simulink model "Speed_control"  (R2023a)
settings: Solver=VariableStepAuto  StartTime=0.0  StopTime=10.0  RelTol=1e-3
libraries: spsMosfetLib x6, simulink x6, spsControlledVoltageSourceLib x1
settings Model: Creator=SIDDHARTHI  LastModifiedBy=SIDDHARTHI

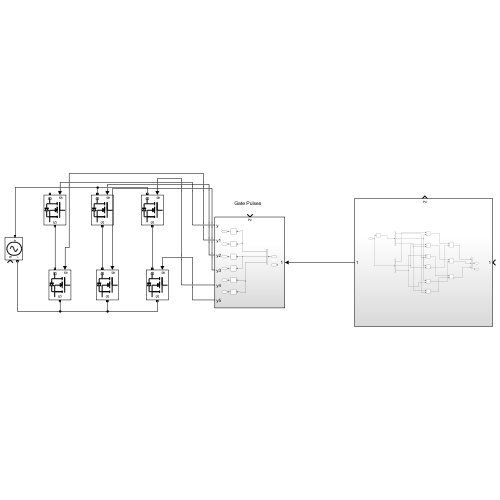
[thumbnail: Simulink's stored preview of the top-level diagram]
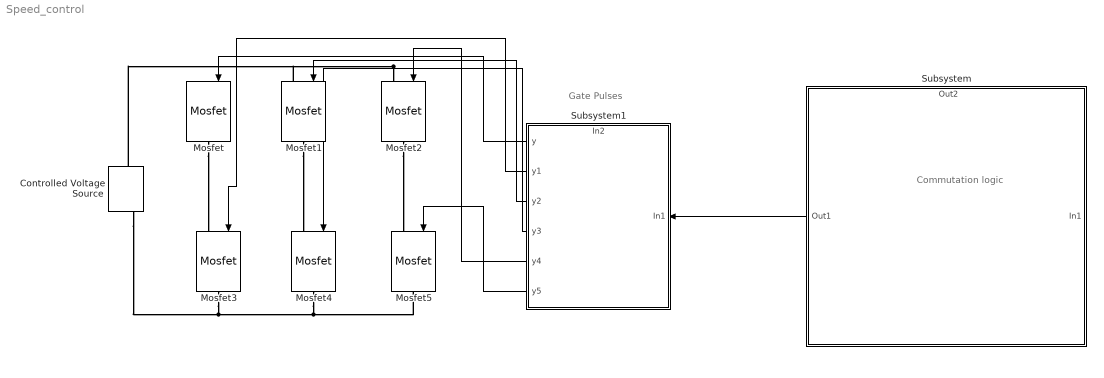
== system Speed_control ==
  note: Gate Pulses
  note: Commutation logic
  Controlled Voltage Source : spsControlledVoltageSourceLib/Controlled Voltage Source  Initialize=on  Source_Type=AC  Amplitude=0  Phase=0  Frequency=0  Measurements=None
  Mosfet{,1..5} (6 alike) : spsMosfetLib/Mosfet  Ron=0.1  Lon=0  Rd=0.01  Vfd=0  IC=0  Rs=1e5  Cs=inf  Measurements=off
  Subsystem : Subsystem
      settings: PortSchema="{\"entries\":[{\"content\":{\"sides\":[{\"content\":{\"connectorIds\":[\"In1\"]},\"type\":\"ConnectorPlacement.EquallySpacedRectSide\",\"uuid\":\"c6f64735-7ac5-4440-9878-dec694729caa\"},{\"content\":{\"connectorIds\":[\"Out1\"],\"side\":\"RIGHT\"},\"type\":\"ConnectorPlacement.EquallySpacedRectSide\",\"uuid\":\"73249ddc-511b-4d67-9c67-fa8b06da8655\"},{\"content\":{\"side\":\"TOP\"},\"type\":\"ConnectorPlacement.EquallySpacedRectSide\",\"uuid\":\"a83625e0-21e7-4ef0-a888-cc1c9f698525\"},{\"content\":{\"connectorIds\":[\"Out2\"],\"side\":\"BOTTOM\"},\"type\":\"ConnectorPlacement.EquallySpacedRectSide\",\"uuid\":\"6631dad1-f62e-4993-8566-3c215e194fd7\"}]},\"type\":\"ConnectorPlacement.EquallySpacedConnector\",\"uuid\":\"77af0196-617d-4c9e-9393-8e6b64813ee3\"}],\"packageUris\":[\"http://schema.mathworks.com/mf0/Connector/R2020b\"],\"version\":\"1.0\"}"
  Subsystem1 : Subsystem
      settings: PortSchema="{\"entries\":[{\"content\":{\"sides\":[{\"content\":{\"connectorIds\":[\"In1\"]},\"type\":\"ConnectorPlacement.EquallySpacedRectSide\",\"uuid\":\"159f6210-f873-4a0a-8ec8-ad944fbd35e4\"},{\"content\":{\"connectorIds\":[\"Out1\",\"Out2\",\"Out3\",\"Out4\",\"Out5\",\"Out6\"],\"side\":\"RIGHT\"},\"type\":\"ConnectorPlacement.EquallySpacedRectSide\",\"uuid\":\"7af34db8-0d64-49dc-873e-7d44036049bf\"},{\"content\":{\"connectorIds\":[\"In2\"],\"side\":\"TOP\"},\"type\":\"ConnectorPlacement.EquallySpacedRectSide\",\"uuid\":\"68cca37c-d2ed-4993-85cf-33e8d45fc75d\"}]},\"type\":\"ConnectorPlacement.EquallySpacedConnector\",\"uuid\":\"7f2c9cee-808d-4302-ab4b-086ba4de1c8b\"}],\"packageUris\":[\"http://schema.mathworks.com/mf0/Connector/R2020b\"],\"version\":\"1.0\"}"
  wires:
  Subsystem/1(Out1) -> Subsystem1/1(In1)
  Subsystem1/1(y) -> Mosfet/1
  Subsystem1/2(y1) -> Mosfet3/1
  Subsystem1/3(y2) -> Mosfet1/1
  Subsystem1/4(y3) -> Mosfet4/1
  Subsystem1/5(y4) -> Mosfet2/1
  Subsystem1/6(y5) -> Mosfet5/1
  connections:
  Mosfet3/RConn1 -- Controlled Voltage Source/LConn1 -- Mosfet4/RConn1 -- Mosfet5/RConn1
  Mosfet/RConn1 -- Mosfet3/LConn1
  Mosfet1/RConn1 -- Mosfet4/LConn1
  Mosfet2/RConn1 -- Mosfet5/LConn1
  Mosfet2/LConn1 -- Controlled Voltage Source/RConn1 -- Mosfet1/LConn1

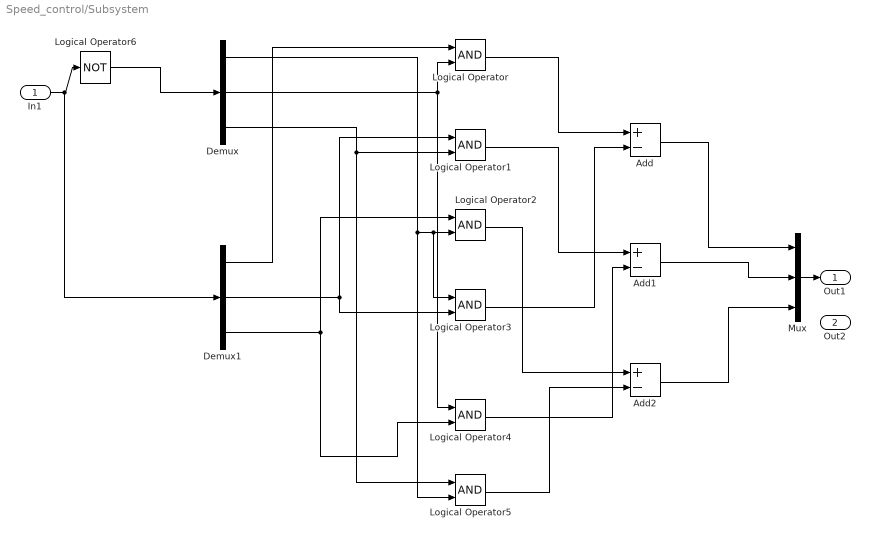
== system Speed_control/Subsystem ==
  In1 : Inport
  Add : Sum  Inputs=+-
  Add1 : Sum  Inputs=+-
  Add2 : Sum  Inputs=+-
  Demux : Demux  Outputs=3
  Demux1 : Demux  Outputs=3
  Logical Operator{,1..5} (6 alike) : Logic  AllPortsSameDT=off  OutDataTypeStr=boolean
  Logical Operator6 : Logic  Operator=NOT  AllPortsSameDT=off  OutDataTypeStr=boolean
  Mux : Mux  Inputs=3
  Out1 : Outport
  Out2 : Outport  Port=2
  wires:
  Demux1/2 -> Logical Operator3/2, Logical Operator1/1
  Add/1 -> Mux/1
  Demux/1 -> Logical Operator5/2, Logical Operator3/1, Logical Operator2/2
  Logical Operator2/1 -> Add2/1
  In1/1 -> Demux1/1, Logical Operator6/1
  Mux/1 -> Out1/1
  Add2/1 -> Mux/3
  Logical Operator5/1 -> Add2/2
  Logical Operator3/1 -> Add/2
  Demux/2 -> Logical Operator/2, Logical Operator4/1
  Demux1/1 -> Logical Operator/1
  Add1/1 -> Mux/2
  Logical Operator/1 -> Add/1
  Logical Operator1/1 -> Add1/1
  Demux1/3 -> Logical Operator4/2, Logical Operator2/1
  Logical Operator4/1 -> Add1/2
  Demux/3 -> Logical Operator5/1, Logical Operator1/2
  Logical Operator6/1 -> Demux/1

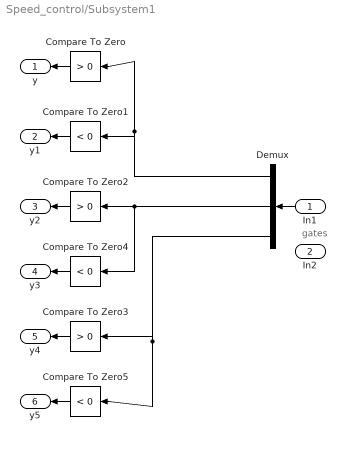
== system Speed_control/Subsystem1 ==
  note: gates
  In1 : Inport
  In2 : Inport  Port=2
  Compare To Zero : simulink/Logic and Bit Operations/Compare To Zero  relop=>  OutDataTypeStr=boolean
  Compare To Zero1 : simulink/Logic and Bit Operations/Compare To Zero  relop=<  OutDataTypeStr=boolean
  Compare To Zero2 : simulink/Logic and Bit Operations/Compare To Zero  relop=>  OutDataTypeStr=boolean
  Compare To Zero3 : simulink/Logic and Bit Operations/Compare To Zero  relop=>  OutDataTypeStr=boolean
  Compare To Zero4 : simulink/Logic and Bit Operations/Compare To Zero  relop=<  OutDataTypeStr=boolean
  Compare To Zero5 : simulink/Logic and Bit Operations/Compare To Zero  relop=<  OutDataTypeStr=boolean
  Demux : Demux  Outputs=3
  y : Outport
  y1 : Outport  Port=2
  y2 : Outport  Port=3
  y3 : Outport  Port=4
  y4 : Outport  Port=5
  y5 : Outport  Port=6
  wires:
  Demux/3 -> Compare To Zero5/1, Compare To Zero3/1
  Compare To Zero/1 -> y/1
  Demux/2 -> Compare To Zero4/1, Compare To Zero2/1
  Demux/1 -> Compare To Zero/1, Compare To Zero1/1
  Compare To Zero5/1 -> y5/1
  Compare To Zero3/1 -> y4/1
  Compare To Zero1/1 -> y1/1
  Compare To Zero4/1 -> y3/1
  In1/1 -> Demux/1
  Compare To Zero2/1 -> y2/1
